simulink model "QUARC_simlink"  (R2023a)
settings: Solver=FixedStepDiscrete  StartTime=0.0  StopTime=inf  FixedStep=0.002  RelTol=1e-3  EnableMultiTasking=on
undefined symbols (not defined in the file or in its folder): HIL
libraries: quarc_library x5
settings Model: ExtModeTrigDuration=10000  Creator=uos  LastModifiedBy=uos
settings SolverCC: AlgebraicLoopSolver=TrustRegion  PositivePriorityOrder=on
settings DataIOCC: ReturnWorkspaceOutputs=off
settings DebuggingCC: UnconnectedInputMsg=warning  UnconnectedOutputMsg=warning  UnconnectedLineMsg=warning  ArithmeticOperatorsInVariantConditions=warning
settings ModelReferenceCC: EnableRefExpFcnMdlSchedulingChecks=on
settings SFSimCC: SimUseLocalCustomCode=off  CustomCodeUndefinedFunction=UseInterfaceOnly
settings RTWCC: Description=QUARC Win64 Target Using Toolchain  SystemTargetFile=quarc_win64.tlc  TemplateMakefile=quarc_default_tmf  RTWUseLocalCustomCode=off  Toolchain=QUARC win64 | nmake (64-bit Windows)  BuildConfiguration=Faster Runs
settings CodeAppCC: StateflowObjectComments=on
settings STFCustomTargetCC: SystemTargetFile=quarc_win64.tlc
settings GRTTargetCC: ParMdlRefBuildCompliant=off  CompOptLevelCompliant=off  CombineOutputUpdateFcns=off  MatFileLogging=off  CPPClassGenCompliant=off  GRTInterface=on  ExtMode=on  ExtModeMexFile=quarc_comm
settings ConfigComp: CovMetricSettings=dswe

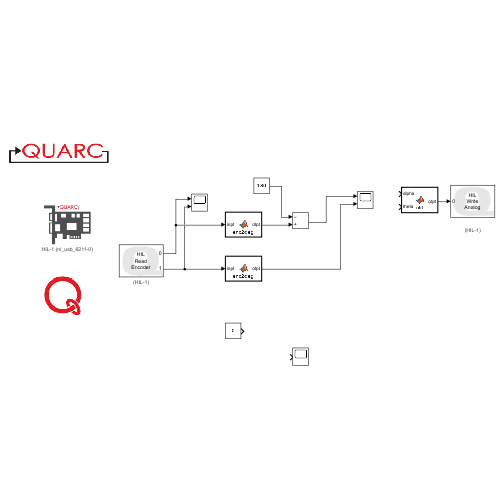
[thumbnail: Simulink's stored preview of the top-level diagram]
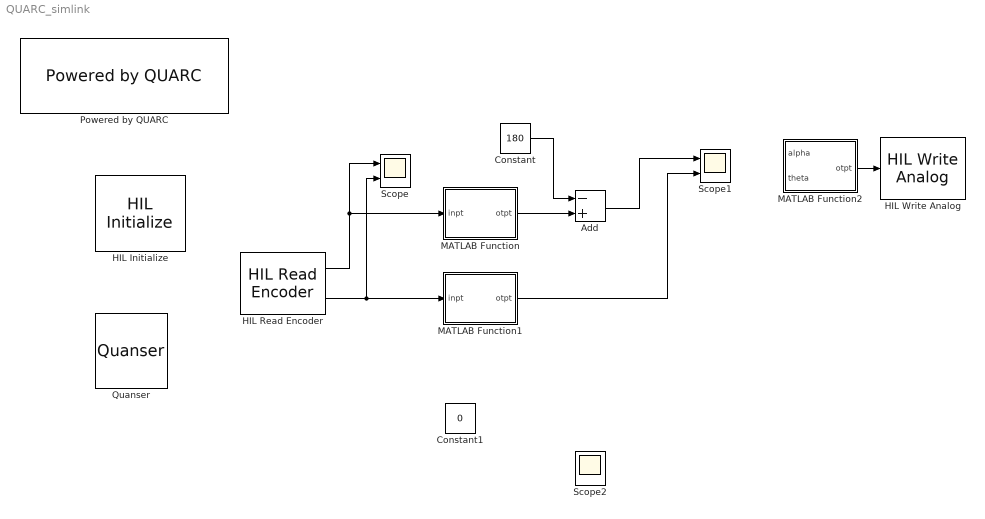
== system QUARC_simlink ==
  Add : Sum  Inputs=-+
  Constant : Constant  Value=180
  Constant1 : Constant  Value=0
  HIL Initialize : quarc_library/Data Acquisition/Generic/Configuration/HIL Initialize  object_name=HIL-1  board_type=ni_usb_6211  board_number=0  board_options=""  exclusive=off  active=on  hardware_clocks=[]  clock_modes=[]  initial_clock_frequencies=[]  set_clock_params_at_start=off  set_clock_params_at_switch_in=off  set_clock_frequencies_at_start=off  set_clock_frequencies_at_switch_in=off  analog_input_channels=[]  analog_input_configurations=[]  analog_input_maximums=10  analog_input_minimums=-10  set_analog_input_params_at_start=on  set_analog_input_params_at_switch_in=off  analog_output_channels=[]  analog_output_maximums=10  analog_output_minimums=-10  initial_analog_outputs=[0]  final_analog_outputs=[0]  watchdog_analog_outputs=[]  set_analog_output_params_at_start=on  set_analog_output_params_at_switch_in=off  set_analog_outputs_at_start=on  set_analog_outputs_at_switch_in=off  set_analog_outputs_at_terminate=on  set_analog_outputs_at_switch_out=off  set_analog_outputs_on_watchdog=off  digital_input_channels=[]  digital_output_channels=[]  digital_output_configuration=[]  initial_digital_outputs=[1]  final_digital_outputs=[1]  watchdog_digital_outputs=[]  set_digital_output_params_at_start=off  set_digital_output_params_at_switch_in=off  set_digital_outputs_at_start=on  set_digital_outputs_at_switch_in=off  set_digital_outputs_at_terminate=on  set_digital_outputs_at_switch_out=off  set_digital_outputs_on_watchdog=off  encoder_channels=[0:1]  quadrature=[4]  encoder_filter_frequency=[]  initial_encoder_counts=[0]  set_encoder_params_at_start=on  set_encoder_params_at_switch_in=off  set_encoder_counts_at_start=on  set_encoder_counts_at_switch_in=on  pwm_channels=[]  pwm_modes=[]  pwm_frequency=80e6/4096  pwm_configuration=[]  pwm_alignment=[]  pwm_polarity=[]  pwm_leading_deadband=[]  pwm_trailing_deadband=[]  initial_pwm_outputs=[0]  final_pwm_outputs=[0]  watchdog_pwm_outputs=[]  set_pwm_params_at_start=on  set_pwm_params_at_switch_in=off  set_pwm_outputs_at_start=on  set_pwm_outputs_at_switch_in=off  set_pwm_outputs_at_terminate=on  set_pwm_outputs_at_switch_out=off  set_pwm_outputs_on_watchdog=off  other_output_channels=[]  initial_other_outputs=[]  final_other_outputs=[]  watchdog_other_outputs=[]  set_other_outputs_at_start=off  set_other_outputs_at_switch_in=off  set_other_outputs_at_terminate=off  set_other_outputs_at_switch_out=off  set_other_outputs_on_watchdog=off
  HIL Read Encoder : quarc_library/Data Acquisition/Generic/Immediate I//O/HIL Read Encoder  object_name=HIL-1  channels=[0:1]  sample_time=qc_get_step_size  active=on  vector_output=off  data_type_mode=Inherit via back propagation  data_type=double
  HIL Write Analog : quarc_library/Data Acquisition/Generic/Immediate I//O/HIL Write Analog  object_name=HIL-1  channels=0  sample_time=-1  active=off  vector_input=off
  MATLAB Function : MATLAB Function  TreatAsAtomicUnit=on
  MATLAB Function1 : MATLAB Function  TreatAsAtomicUnit=on
  MATLAB Function2 : MATLAB Function  TreatAsAtomicUnit=on
  Powered by QUARC : quarc_library/Logos/Powered by QUARC
  Quanser : quarc_library/Logos/Quanser
  Scope : Scope  NumInputPorts=2
  Scope1 : Scope  NumInputPorts=2
  Scope2 : Scope
  wires:
  HIL Read Encoder/1 -> Scope/1, MATLAB Function/1(inpt)
  HIL Read Encoder/2 -> MATLAB Function1/1(inpt), Scope/2
  MATLAB Function/1(otpt) -> Add/2
  Constant/1 -> Add/1
  Add/1 -> Scope1/1
  MATLAB Function1/1(otpt) -> Scope1/2
  MATLAB Function2/1(otpt) -> HIL Write Analog/1

== matlab function QUARC_simlink/MATLAB Function ==
  data: inpt input; otpt output
function otpt  = enc2deg(inpt)
%ENC2DEG converts raw encnder readings to degreess. it handles wraparound +
%conversion. 

%constants 
encoderCPR = 4096;
conterBits = 32; 

%remove wraparound 
wraparoundThresh = 2^(conterBits-1);
inpt(inpt > wraparoundThresh) = inpt(inpt > wraparoundThresh) - 2^conterBits;

%convert to deg 
otpt = inpt*360/encoderCPR;
end

== matlab function QUARC_simlink/MATLAB Function2 ==
  data: alpha input; otpt output; theta input
function otpt  = ctrl(alpha,theta)
%ENC2DEG converts raw encnder readings to degreess. it handles wraparound +
%conversion. 

%constants 
encoderCPR = 4096;
conterBits = 32; 

%remove wraparound 
wraparoundThresh = 2^(conterBits-1);
inpt(inpt > wraparoundThresh) = inpt(inpt > wraparoundThresh) - 2^conterBits;

%convert to deg 
otpt = inpt*360/encoderCPR;
end

== matlab function QUARC_simlink/MATLAB Function1 ==
  data: inpt input; otpt output
function otpt  = enc2deg(inpt)
%ENC2DEG converts raw encnder readings to degreess. it handles wraparound +
%conversion. 

%constants 
encoderCPR = 4096;
conterBits = 32; 

%remove wraparound 
wraparoundThresh = 2^(conterBits-1);
inpt(inpt > wraparoundThresh) = inpt(inpt > wraparoundThresh) - 2^conterBits;

%convert to deg 
otpt = inpt*360/encoderCPR;
end
